simulink model "exnb4137986_Q4"  (R2024b)
settings: Solver=FixedStepAuto  StartTime=0.0  StopTime=15  FixedStep=0.001  RelTol=1e-3
values from neighbouring files (symbols this model uses):
  m_star_1 = double(subs(m, x2, omega_star_1))    [exnb4137986_Q4_par.m]    (also in exnb4137986_Q6_par.m; exnb4137986_Q8_par.m; exnb4137986_Q9_par.m)
  m_star_2 = double(subs(m, x2, omega_star_2))    [exnb4137986_Q4_par.m]    (also in exnb4137986_Q6_par.m; exnb4137986_Q8_par.m; exnb4137986_Q9_par.m)
  omega_star_1 = 200    [exnb4137986_Q4_par.m]    (also in exnb4137986_Q6_par.m; exnb4137986_Q8_par.m; exnb4137986_Q9_par.m)
  omega_star_2 = 300    [exnb4137986_Q4_par.m]    (also in exnb4137986_Q6_par.m; exnb4137986_Q8_par.m; exnb4137986_Q9_par.m)
  u_star_1 = double(subs(u, x2, omega_star_1))    [exnb4137986_Q4_par.m]    (also in exnb4137986_Q6_par.m; exnb4137986_Q8_par.m; exnb4137986_Q9_par.m)
  values = [1, 10, 0.1, 40]    [exnb4137986_Q4_par.m]    (also in exnb4137986_Q6_par.m; exnb4137986_Q8_par.m; exnb4137986_Q9_par.m)
settings Model: Creator=therkelsen  LastModifiedBy=therkelsen

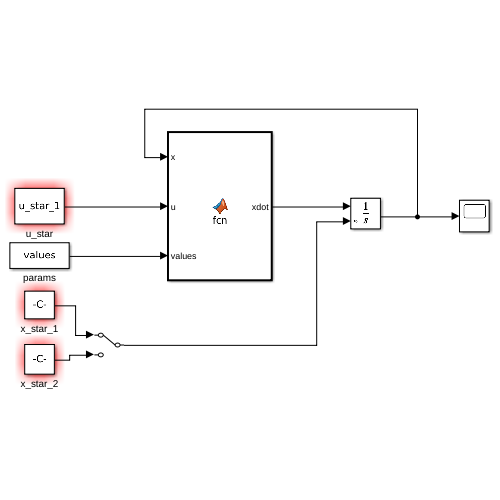
[thumbnail: Simulink's stored preview of the top-level diagram]
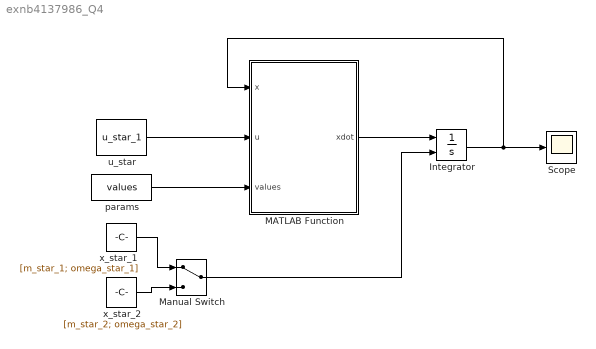
== system exnb4137986_Q4 ==
  Integrator : Integrator  InitialConditionSource=external
  MATLAB Function : MATLAB Function  TreatAsAtomicUnit=on
  Manual Switch : ManualSwitch
  Scope : Scope
  params : Constant  Value=values
  u_star : Constant  Value=u_star_1
  x_star_1 : Constant  Value=[m_star_1; omega_star_1]
  x_star_2 : Constant  Value=[m_star_2; omega_star_2]
  wires:
  params/1 -> MATLAB Function/3(values)
  MATLAB Function/1(xdot) -> Integrator/1
  Integrator/1 -> Scope/1, MATLAB Function/1(x)
  Manual Switch/1 -> Integrator/2
  u_star/1 -> MATLAB Function/2(u)
  x_star_1/1 -> Manual Switch/1
  x_star_2/1 -> Manual Switch/2

== matlab function exnb4137986_Q4/MATLAB Function ==
  data: x input; u input; xdot output; values input
function xdot = fcn(x, u, values)

q1 = values(1);
q2 = values(2);
q3 = values(3);
J = values(4);

xdot = [-q1*x(2)*x(1) + u;
         q2/J*x(1) - q3/J*x(2)];
